simulink model "Full_Model_D_R2"  (R2013a)
settings: Solver=ode45  StartTime=0.0  StopTime=sim_length  MaxStep=1e-4  RelTol=1e-3
values from neighbouring files (symbols this model uses):
  B = 0    [Model_Parameters.mat]
  D = 4.45306861536e-07    [Model_Parameters.mat]
  F_yIntercept = -10.4432883127    [Model_Parameters.mat]
  Feed_Forward_Yaw_d = 0    [Yaw_Controller_SS_D_Data.mat]
  g = 9.81    [Model_Parameters.mat]
  I_Phi = I_Gamma    [Main_Controller_Test_C.m]
  I_Psi = 0.236966962973    [Model_Parameters.mat]
  I_Theta = 0.127422725814    [Model_Parameters.mat]
  J = 8e-08    [Model_Parameters.mat]
  Kf = 9.48907430341    [Model_Parameters.mat]
  Kw = 501.513336009    [Model_Parameters.mat]
  L = 0.338    [Model_Parameters.mat]
  Mass = 2.26    [Model_Parameters.mat]
  Motor_TimeConstant = 0.07    [Model_Parameters.mat]
  omega_0 = (5.6-F_yIntercept)/Kf    [Main_Controller_Test_C.m]
  omega_Lim = (0-F_yIntercept)/Kf    [Main_Controller_Test_C.m]
  Phi_IC = (2/180)*pi    (= 0.0349065850399)    [Main_Controller_Test_C.m]
  Pitch_Setpoint = 0    [Main_Controller_Test_C.m]
  Psi_IC = (10/180)*pi    (= 0.174532925199)    [Main_Controller_Test_C.m]
  PWM_IC = 1.4    [Main_Controller_Test_C.m]
  Speed_yIntercept = -347.939581678    [Model_Parameters.mat]
  Theta_IC = (2/180)*pi    (= 0.0349065850399)    [Main_Controller_Test_C.m]
  Yaw_Setpoint = 0    [Main_Controller_Test_C.m]
undefined symbols (not defined in the file or in its folder): DiscIntNeverNeededParam, Feed_Forward_Roll_d, Ts
libraries: simulink x6
settings Model: Creator=Ross  LastModifiedBy=Ross

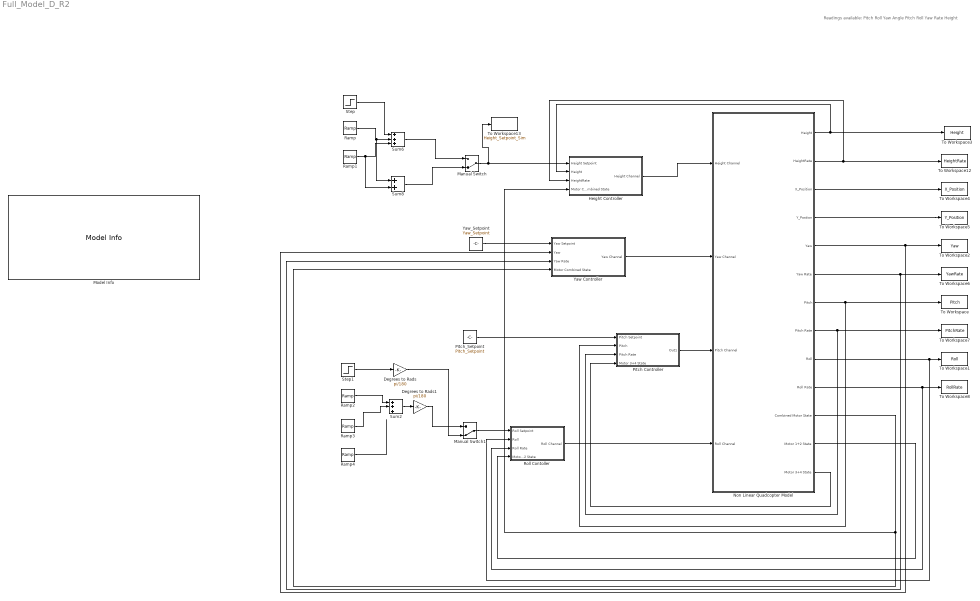
== system Full_Model_D_R2 ==
  note: Readings available:
      | Pitch Roll Yaw Angle
      | Pitch Roll Yaw Rate
      | Height
  Degrees to Rads : Gain  Gain=pi/180
  Degrees to Rads1 : Gain  Gain=pi/180
  Height Controller : Subsystem
  Manual Switch : ManualSwitch  CurrentSetting=0
  Manual Switch1 : ManualSwitch  CurrentSetting=0
  Model Info : simulink/Model-Wide Utilities/Model Info  InitialBlockCM=None  BlockCM=None  Frame=on  DisplayStringWithTags=|  HorizontalTextAlignment=Center  LeftAlignmentValue=0.5  SourceBlockDiagram=Full_Model_D_R2  TagMaxNumber=20
      | %<ModelName>
      | Simulink Diagram Used in Testing of Controllers designed for Quadcopters
      | Model version is %<ModelVersion>
      | 
      | %<Created>
      | %<ModifiedBy>
      | %<ModifiedDate>
      | %<ModifiedComment>
      | 
      | 
      | %<LastModifiedBy>
      | %<LastModificationDate>
      | %<Description>
  Non Linear Quadcopter Model : Subsystem
  Pitch Controller : Subsystem
  "Pitch_Setpoint " : Constant  Value=Pitch_Setpoint
  Ramp : simulink/Sources/Ramp  slope=1  start=2  X0=0
  Ramp1 : simulink/Sources/Ramp  slope=-1  start=5  X0=0
  Ramp2 : simulink/Sources/Ramp  slope=20  start=10  X0=0
  Ramp3 : simulink/Sources/Ramp  slope=-10  start=11  X0=0
  Ramp4 : simulink/Sources/Ramp  slope=2  start=22  X0=0
  Roll Contoller : Subsystem
  Step : Step  Time=10  SampleTime=0
  Step1 : Step  Time=12  After=40  SampleTime=0
  Sum2 : Sum  Inputs=+++
  Sum6 : Sum  Inputs=+++
  Sum8 : Sum
  To Workspace : ToWorkspace  VariableName=Pitch  SampleTime=-1  SaveFormat=Timeseries
  To Workspace1 : ToWorkspace  VariableName=Roll  SampleTime=-1  SaveFormat=Timeseries
  To Workspace12 : ToWorkspace  VariableName=HeightRate  SampleTime=-1  SaveFormat=Timeseries
  To Workspace13 : ToWorkspace  VariableName=Height_Setpoint_Sim  SampleTime=-1  SaveFormat=Timeseries
  To Workspace2 : ToWorkspace  VariableName=Yaw  SampleTime=-1  SaveFormat=Timeseries
  To Workspace3 : ToWorkspace  VariableName=Height  SampleTime=-1  SaveFormat=Timeseries
  To Workspace4 : ToWorkspace  VariableName=X_Position  SampleTime=-1  SaveFormat=Timeseries
  To Workspace5 : ToWorkspace  VariableName=Y_Position  SampleTime=-1  SaveFormat=Timeseries
  To Workspace6 : ToWorkspace  VariableName=YawRate  SampleTime=-1  SaveFormat=Timeseries
  To Workspace7 : ToWorkspace  VariableName=PitchRate  SampleTime=-1  SaveFormat=Timeseries
  To Workspace8 : ToWorkspace  VariableName=RollRate  SampleTime=-1  SaveFormat=Timeseries
  Yaw Controller : Subsystem
  Yaw_Setpoint : Constant  Value=Yaw_Setpoint
  wires:
  Non Linear Quadcopter Model/5(Yaw) -> Yaw Controller/2(Yaw), To Workspace2/1
  Non Linear Quadcopter Model/1(Height) -> To Workspace3/1, Height Controller/2(Height)
  Non Linear Quadcopter Model/3(X_Position) -> To Workspace4/1
  Non Linear Quadcopter Model/4(Y_Postion) -> To Workspace5/1
  Non Linear Quadcopter Model/6(Yaw Rate) -> Yaw Controller/3(Yaw Rate), To Workspace6/1
  Non Linear Quadcopter Model/8(Pitch Rate) -> Pitch Controller/3(Pitch Rate), To Workspace7/1
  Non Linear Quadcopter Model/10(Roll Rate) -> To Workspace8/1, Roll Contoller/3(Roll Rate)
  Ramp/1 -> Sum8/1, Sum6/2
  Ramp1/1 -> Sum8/2, Sum6/3
  Step/1 -> Sum6/1
  Manual Switch/1 -> Height Controller/1(Height Setpoint), To Workspace13/1
  Sum8/1 -> Manual Switch/2
  Sum6/1 -> Manual Switch/1
  Non Linear Quadcopter Model/9(Roll) -> To Workspace1/1, Roll Contoller/2(Roll)
  Non Linear Quadcopter Model/7(Pitch) -> Pitch Controller/2(Pitch), To Workspace/1
  Ramp2/1 -> Sum2/1
  Ramp3/1 -> Sum2/2
  Step1/1 -> Degrees to Rads/1
  Sum2/1 -> Degrees to Rads1/1
  Degrees to Rads/1 -> Manual Switch1/2
  "Pitch_Setpoint "/1 -> Pitch Controller/1(Pitch Setpoint)
  Non Linear Quadcopter Model/13(Motor 3+4 State) -> Pitch Controller/4(Motor 3+4 State)
  Pitch Controller/1(Out1) -> Non Linear Quadcopter Model/3(Pitch Channel)
  Manual Switch1/1 -> Roll Contoller/1("Roll Setpoint ")
  Non Linear Quadcopter Model/12(Motor 1+2 State) -> Roll Contoller/4(Motor 1+2 State)
  Roll Contoller/1(Roll Channel) -> Non Linear Quadcopter Model/4(Roll Channel)
  Yaw_Setpoint/1 -> Yaw Controller/1(Yaw Setpoint)
  Yaw Controller/1(Yaw Channel) -> Non Linear Quadcopter Model/2(Yaw Channel)
  Height Controller/1(Height Channel) -> Non Linear Quadcopter Model/1(Height Channel)
  Non Linear Quadcopter Model/2(HeightRate) -> Height Controller/3(HeightRate), To Workspace12/1
  Non Linear Quadcopter Model/11(Combined Motor State) -> Height Controller/4(Motor Combined State), Yaw Controller/4(Motor Combined State)
  Degrees to Rads1/1 -> Manual Switch1/1
  Ramp4/1 -> ?

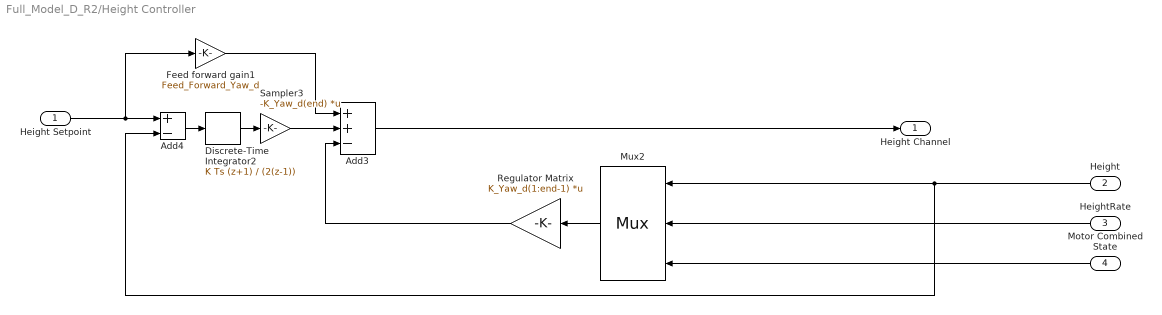
== system Full_Model_D_R2/Height Controller ==
  Height Setpoint : Inport
  Height : Inport  Port=2
  HeightRate : Inport  Port=3
  Motor Combined State : Inport  Port=4
  Add3 : Sum  Inputs=++-
  Add4 : Sum  Inputs=+-  SampleTime=Ts
  Discrete-Time Integrator2 : DiscreteIntegrator  IntegratorMethod=Integration: Trapezoidal  gainval=1  InitialCondition=PWM_IC  SampleTime=Ts  ICPrevOutput=DiscIntNeverNeededParam  ICPrevScaledInput=DiscIntNeverNeededParam
  Feed forward gain1 : Gain  Gain=Feed_Forward_Yaw_d  SampleTime=Ts
  Mux2 : Mux  Inputs=3
      settings: DisplayOption=signals
  Regulator Matrix : Gain  Gain=K_Yaw_d(1:end-1)  Multiplication=Matrix(K*u)  SampleTime=Ts
  Sampler3 : Gain  Gain=-K_Yaw_d(end)  Multiplication=Matrix(K*u)  SampleTime=Ts
  Height Channel : Outport
  wires:
  Height/1 -> Add4/2, Mux2/1
  Feed forward gain1/1 -> Add3/1
  Add3/1 -> Height Channel/1
  Motor Combined State/1 -> Mux2/3
  Mux2/1 -> Regulator Matrix/1
  Regulator Matrix/1 -> Add3/3
  Add4/1 -> Discrete-Time Integrator2/1
  Discrete-Time Integrator2/1 -> Sampler3/1
  Sampler3/1 -> Add3/2
  Height Setpoint/1 -> Feed forward gain1/1, Add4/1
  HeightRate/1 -> Mux2/2

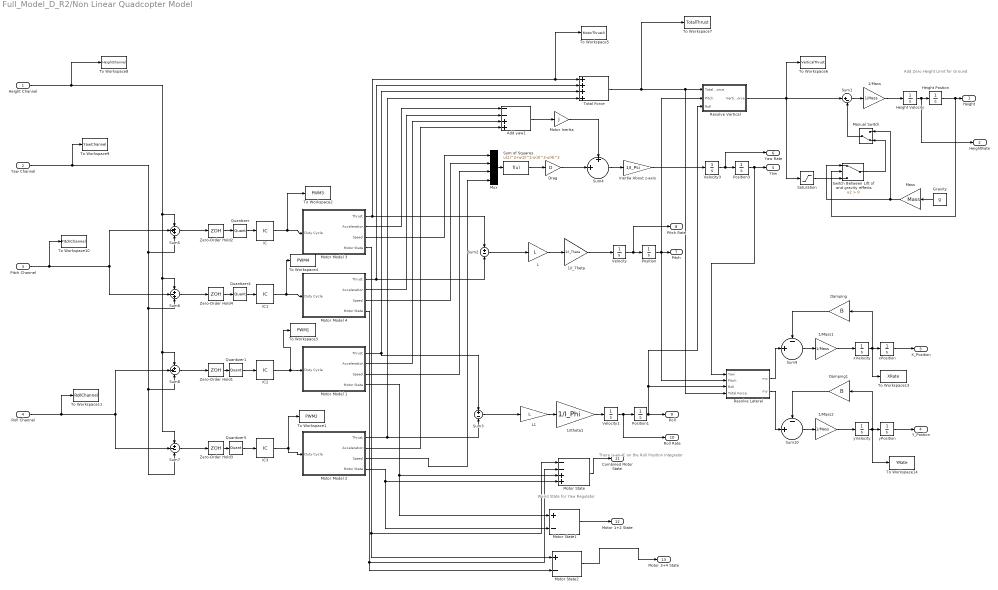
== system Full_Model_D_R2/Non Linear Quadcopter Model ==
  note: Weird State for Yaw
      | Regulator
  note: There is an IC on the Roll
      | Position Integrator
  note: Add Zero Height Limit
      | for Ground
  Height Channel : Inport
  Yaw Channel : Inport  Port=2
  Pitch Channel : Inport  Port=3
  Roll Channel : Inport  Port=4
  1/I_Theta : Gain  Gain=1/I_Theta
  1/Itheta1 : Gain  Gain=1/I_Phi
  1/Mass : Gain  Gain=1/Mass
  1/Mass1 : Gain  Gain=1/Mass
  1/Mass2 : Gain  Gain=1/Mass
  Add yaw1 : Sum  Inputs=--++
  Damping : Gain  Gain=B
  Damping1 : Gain  Gain=B
  Drag : Gain  Gain=D
  Gravity : Constant  Value=g
  Height Postion : Integrator  LowerSaturationLimit=0
  Height Velocity : Integrator
  IC{,1..3} (4 alike) : InitialCondition
  Inertia About z-axis : Gain  Gain=1/I_Psi
  L : Gain  Gain=L
  L1 : Gain  Gain=L
  Manual Switch : ManualSwitch  CurrentSetting=0
  Mass : Gain  Gain=Mass
  Motor Inertia : Gain  Gain=J
  Motor Model 1 : Subsystem
  Motor Model 2 : Subsystem
  Motor Model 3 : Subsystem
  Motor Model 4 : Subsystem
  Motor State : Sum  Inputs=--++
  Motor State1 : Sum  Inputs=+-
  Motor State2 : Sum  Inputs=+-
  Mux : Mux
  Position : Integrator  InitialCondition=Theta_IC
  Position1 : Integrator  InitialCondition=Phi_IC
  Position3 : Integrator  InitialCondition=Psi_IC
  Quantizer{,1,4..5} (4 alike) : Quantizer  QuantizationInterval=8.2e-3
  Resolve Lateral : Subsystem
  Resolve Vertical : Subsystem
  Saturation : Saturate  UpperLimit=Mass*g  LowerLimit=-inf
  Sum of Squares : Fcn  Expr=u(1)^2+u(2)^2-u(3)^2-u(4)^2
  Sum1 : Sum  Inputs=|+-
  Sum10 : Sum  Inputs=-|||+||||
  Sum2 : Sum  Inputs=+|-
  Sum3 : Sum  Inputs=+|-
  Sum4 : Sum  Inputs=+|||+||||
  Sum5 : Sum  Inputs=+++
  Sum6 : Sum  Inputs=+-+
  Sum7 : Sum  Inputs=+--
  Sum8 : Sum  Inputs=++-
  Sum9 : Sum  Inputs=-|||+||||
  Switch Between Lift of and gravity effects : Switch  Criteria=u2 > Threshold
  To Workspace1 : ToWorkspace  VariableName=PWM2  SampleTime=-1  SaveFormat=Timeseries
  To Workspace10 : ToWorkspace  VariableName=PitchChannel  SampleTime=-1  SaveFormat=Timeseries
  To Workspace11 : ToWorkspace  VariableName=RollChannel  SampleTime=-1  SaveFormat=Timeseries
  To Workspace13 : ToWorkspace  VariableName=XRate  SampleTime=-1  SaveFormat=Timeseries
  To Workspace14 : ToWorkspace  VariableName=YRate  SampleTime=-1  SaveFormat=Timeseries
  To Workspace2 : ToWorkspace  VariableName=PWM3  SampleTime=-1  SaveFormat=Timeseries
  To Workspace3 : ToWorkspace  VariableName=PWM1  SampleTime=-1  SaveFormat=Timeseries
  To Workspace4 : ToWorkspace  VariableName=PWM4  SampleTime=-1  SaveFormat=Timeseries
  To Workspace5 : ToWorkspace  VariableName=MotorThrust3  SampleTime=-1  SaveFormat=Timeseries
  To Workspace6 : ToWorkspace  VariableName=VerticalThrust  SampleTime=-1  SaveFormat=Timeseries
  To Workspace7 : ToWorkspace  VariableName=TotalThrust  SampleTime=-1  SaveFormat=Timeseries
  To Workspace8 : ToWorkspace  VariableName=HeightChannel  SampleTime=-1  SaveFormat=Timeseries
  To Workspace9 : ToWorkspace  VariableName=YawChannel  SampleTime=-1  SaveFormat=Timeseries
  Total Force : Sum  Inputs=++++
  Velocity : Integrator
  Velocity1 : Integrator
  Velocity3 : Integrator
  Zero-Order Hold{1..4} (4 alike) : ZeroOrderHold  SampleTime=Ts
  xPosition : Integrator
  xVelocity : Integrator
  yPosition : Integrator
  yVelocity : Integrator
  Height : Outport
  HeightRate : Outport  Port=2
  X_Position : Outport  Port=3
  Y_Postion : Outport  Port=4
  Yaw : Outport  Port=5
  Yaw Rate : Outport  Port=6
  Pitch : Outport  Port=7
  Pitch Rate : Outport  Port=8
  Roll : Outport  Port=9
  Roll Rate : Outport  Port=10
  Combined Motor State : Outport  Port=11
  Motor 1+2 State : Outport  Port=12
  Motor 3+4 State : Outport  Port=13
  wires:
  Sum1/1 -> 1/Mass/1
  Pitch Channel/1 -> Sum6/2, Sum5/2, To Workspace10/1
  Add yaw1/1 -> Motor Inertia/1
  1/Mass/1 -> Height Velocity/1
  Motor Inertia/1 -> Sum4/1
  1/Mass1/1 -> xVelocity/1
  Sum9/1 -> 1/Mass1/1
  xPosition/1 -> X_Position/1
  Damping/1 -> Sum9/1
  xVelocity/1 -> To Workspace13/1, Damping/1, xPosition/1
  Motor Model 3/2(Acceleration) -> Add yaw1/1
  Height Velocity/1 -> HeightRate/1, Height Postion/1
  Sum2/1 -> L/1
  1/I_Theta/1 -> Velocity/1
  Velocity/1 -> Pitch Rate/1, Position/1
  Position/1 -> Resolve Vertical/2(Pitch), Pitch/1, Resolve Lateral/2(Pitch)
  Total Force/1 -> To Workspace7/1, Resolve Lateral/4(Total Force), Resolve Vertical/1(Total Force)
  Sum of Squares/1 -> Drag/1
  Drag/1 -> Sum4/2
  Position3/1 -> Yaw/1, Resolve Lateral/1(Yaw)
  Velocity3/1 -> Yaw Rate/1, Position3/1
  Inertia About z-axis/1 -> Velocity3/1
  Motor Model 2/1(Thrust) -> Total Force/4, Sum3/2
  L1/1 -> 1/Itheta1/1
  Velocity1/1 -> Roll Rate/1, Position1/1
  Sum3/1 -> L1/1
  Position1/1 -> Roll/1, Resolve Lateral/3(Roll), Resolve Vertical/3(Roll)
  1/Itheta1/1 -> Velocity1/1
  Motor Model 3/1(Thrust) -> Sum2/1, To Workspace5/1, Total Force/1
  Sum10/1 -> 1/Mass2/1
  1/Mass2/1 -> yVelocity/1
  yPosition/1 -> Y_Postion/1
  Damping1/1 -> Sum10/1
  yVelocity/1 -> Damping1/1, To Workspace14/1, yPosition/1
  Height Postion/1 -> Switch Between Lift of and gravity effects/2, Height/1
  Motor Model 1/2(Acceleration) -> Add yaw1/3
  Motor Model 4/1(Thrust) -> Sum2/2, Total Force/2
  Sum4/1 -> Inertia About z-axis/1
  Motor Model 1/1(Thrust) -> Sum3/1, Total Force/3
  Height Channel/1 -> To Workspace8/1, Sum6/1, Sum7/1, Sum8/1, Sum5/1
  Yaw Channel/1 -> To Workspace9/1, Sum7/3, Sum8/3, Sum6/3, Sum5/3
  Motor Model 4/2(Acceleration) -> Add yaw1/2
  Motor Model 2/2(Acceleration) -> Add yaw1/4
  Roll Channel/1 -> To Workspace11/1, Sum8/2, Sum7/2
  Gravity/1 -> Mass/1
  Resolve Lateral/1(mx) -> Sum9/2
  Resolve Lateral/2(my) -> Sum10/2
  Motor Model 3/3(Speed) -> Mux/1
  Motor Model 4/3(Speed) -> Mux/2
  Motor Model 1/3(Speed) -> Mux/3
  Motor Model 2/3(Speed) -> Mux/4
  Mux/1 -> Sum of Squares/1
  L/1 -> 1/I_Theta/1
  Switch Between Lift of and gravity effects/1 -> Manual Switch/2
  Saturation/1 -> Switch Between Lift of and gravity effects/3
  Mass/1 -> Manual Switch/1, Switch Between Lift of and gravity effects/1
  Manual Switch/1 -> Sum1/2
  Motor Model 3/4(Motor State) -> Motor State2/1, Motor State/1
  Motor Model 4/4(Motor State) -> Motor State2/2, Motor State/2
  Motor Model 1/4(Motor State) -> Motor State1/1, Motor State/3
  Motor Model 2/4(Motor State) -> Motor State1/2, Motor State/4
  Motor State/1 -> Combined Motor State/1
  Motor State1/1 -> Motor 1+2 State/1
  Motor State2/1 -> Motor 3+4 State/1
  Resolve Vertical/1(Vertical Force) -> Sum1/1, Saturation/1, To Workspace6/1
  Zero-Order Hold2/1 -> Quantizer/1
  Zero-Order Hold1/1 -> Quantizer1/1
  Zero-Order Hold3/1 -> Quantizer5/1
  Zero-Order Hold4/1 -> Quantizer4/1
  IC1/1 -> To Workspace4/1, Motor Model 4/1(Duty Cycle)
  IC2/1 -> To Workspace3/1, Motor Model 1/1(Duty Cycle)
  IC3/1 -> Motor Model 2/1(Duty Cycle), To Workspace1/1
  IC/1 -> To Workspace2/1, Motor Model 3/1(Duty Cycle)
  Sum5/1 -> Zero-Order Hold2/1
  Sum6/1 -> Zero-Order Hold4/1
  Sum8/1 -> Zero-Order Hold1/1
  Sum7/1 -> Zero-Order Hold3/1
  Quantizer/1 -> IC/1
  Quantizer4/1 -> IC1/1
  Quantizer1/1 -> IC2/1
  Quantizer5/1 -> IC3/1

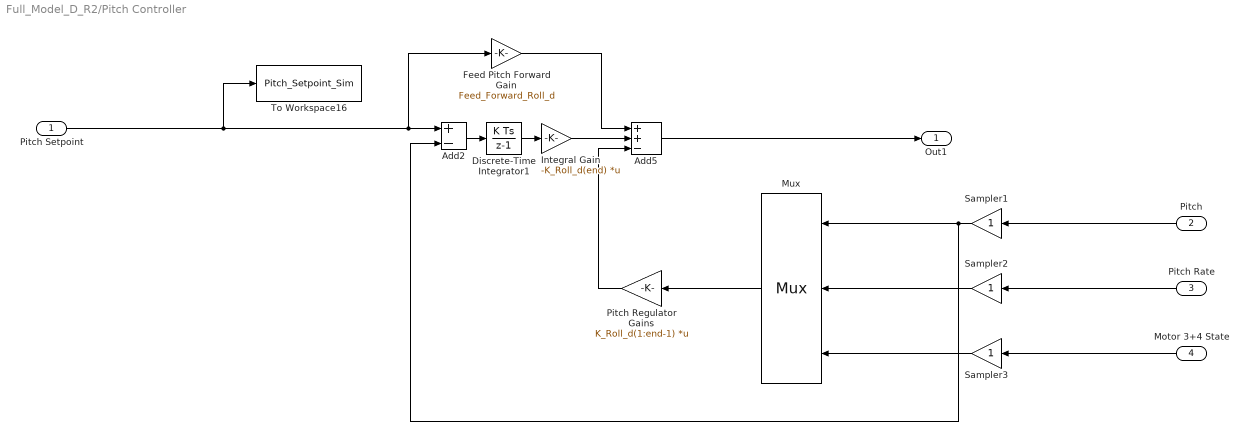
== system Full_Model_D_R2/Pitch Controller ==
  Pitch Setpoint : Inport
  Pitch : Inport  Port=2
  Pitch Rate : Inport  Port=3
  Motor 3+4 State : Inport  Port=4
  Add2 : Sum  Inputs=+-
  Add5 : Sum  Inputs=++-
  Discrete-Time Integrator1 : DiscreteIntegrator  gainval=1  InitialCondition=PWM_IC  SampleTime=Ts  ICPrevOutput=DiscIntNeverNeededParam  ICPrevScaledInput=DiscIntNeverNeededParam
  Feed Pitch Forward Gain : Gain  Gain=Feed_Forward_Roll_d  SampleTime=Ts
  Integral Gain : Gain  Gain=-K_Roll_d(end)  Multiplication=Matrix(K*u)  SampleTime=Ts
  Mux : Mux  Inputs=3
      settings: DisplayOption=signals
  Pitch Regulator Gains : Gain  Gain=K_Roll_d(1:end-1)  Multiplication=Matrix(K*u)
  Sampler1 : Gain  SampleTime=Ts
  Sampler2 : Gain  SampleTime=Ts
  Sampler3 : Gain  SampleTime=Ts
  To Workspace16 : ToWorkspace  VariableName=Pitch_Setpoint_Sim  SampleTime=-1  SaveFormat=Timeseries
  Out1 : Outport
  wires:
  Integral Gain/1 -> Add5/2
  Sampler1/1 -> Add2/2, Mux/1
  Pitch Setpoint/1 -> To Workspace16/1, Feed Pitch Forward Gain/1, Add2/1
  Sampler2/1 -> Mux/2
  Discrete-Time Integrator1/1 -> Integral Gain/1
  Add2/1 -> Discrete-Time Integrator1/1
  Sampler3/1 -> Mux/3
  Add5/1 -> Out1/1
  Mux/1 -> Pitch Regulator Gains/1
  Pitch Regulator Gains/1 -> Add5/3
  Motor 3+4 State/1 -> Sampler3/1
  Feed Pitch Forward Gain/1 -> Add5/1
  Pitch Rate/1 -> Sampler2/1
  Pitch/1 -> Sampler1/1

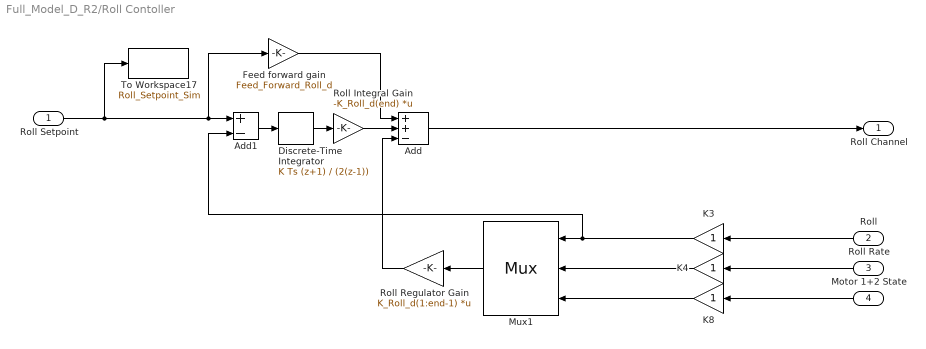
== system Full_Model_D_R2/Roll Contoller ==
  "Roll Setpoint " : Inport
  Roll : Inport  Port=2
  Roll Rate : Inport  Port=3
  Motor 1+2 State : Inport  Port=4
  Add : Sum  Inputs=++-
  Add1 : Sum  Inputs=+-
  Discrete-Time Integrator : DiscreteIntegrator  IntegratorMethod=Integration: Trapezoidal  gainval=1  InitialCondition=PWM_IC  SampleTime=Ts  ICPrevOutput=DiscIntNeverNeededParam  ICPrevScaledInput=DiscIntNeverNeededParam
  Feed forward gain : Gain  Gain=Feed_Forward_Roll_d  SampleTime=Ts
  K3 : Gain  SampleTime=Ts
  K4 : Gain  SampleTime=Ts
  K8 : Gain  SampleTime=Ts
  Mux1 : Mux  Inputs=3
      settings: DisplayOption=signals
  Roll Integral Gain : Gain  Gain=-K_Roll_d(end)  Multiplication=Matrix(K*u)  SampleTime=Ts
  Roll Regulator Gain : Gain  Gain=K_Roll_d(1:end-1)  Multiplication=Matrix(K*u)
  To Workspace17 : ToWorkspace  VariableName=Roll_Setpoint_Sim  SampleTime=-1  SaveFormat=Timeseries
  Roll Channel : Outport
  wires:
  Roll/1 -> K3/1
  K4/1 -> Mux1/2
  K8/1 -> Mux1/3
  Add1/1 -> Discrete-Time Integrator/1
  Discrete-Time Integrator/1 -> Roll Integral Gain/1
  Roll Integral Gain/1 -> Add/2
  K3/1 -> Add1/2, Mux1/1
  "Roll Setpoint "/1 -> Feed forward gain/1, Add1/1, To Workspace17/1
  Feed forward gain/1 -> Add/1
  Roll Regulator Gain/1 -> Add/3
  Mux1/1 -> Roll Regulator Gain/1
  Motor 1+2 State/1 -> K8/1
  Add/1 -> Roll Channel/1
  Roll Rate/1 -> K4/1

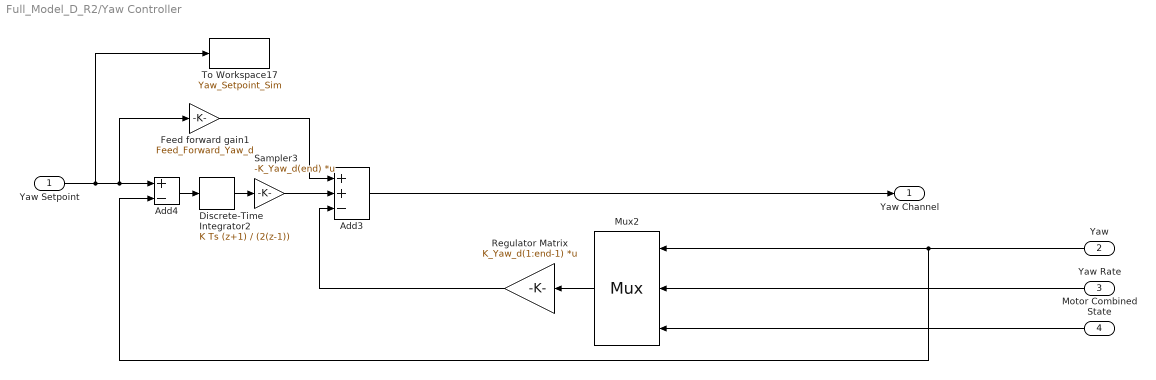
== system Full_Model_D_R2/Yaw Controller ==
  Yaw Setpoint : Inport
  Yaw : Inport  Port=2
  Yaw Rate : Inport  Port=3
  Motor Combined State : Inport  Port=4
  Add3 : Sum  Inputs=++-
  Add4 : Sum  Inputs=+-  SampleTime=Ts
  Discrete-Time Integrator2 : DiscreteIntegrator  IntegratorMethod=Integration: Trapezoidal  gainval=1  InitialCondition=PWM_IC  SampleTime=Ts  ICPrevOutput=DiscIntNeverNeededParam  ICPrevScaledInput=DiscIntNeverNeededParam
  Feed forward gain1 : Gain  Gain=Feed_Forward_Yaw_d  SampleTime=Ts
  Mux2 : Mux  Inputs=3
      settings: DisplayOption=signals
  Regulator Matrix : Gain  Gain=K_Yaw_d(1:end-1)  Multiplication=Matrix(K*u)  SampleTime=Ts
  Sampler3 : Gain  Gain=-K_Yaw_d(end)  Multiplication=Matrix(K*u)  SampleTime=Ts
  To Workspace17 : ToWorkspace  VariableName=Yaw_Setpoint_Sim  SampleTime=-1  SaveFormat=Timeseries
  Yaw Channel : Outport
  wires:
  Yaw/1 -> Add4/2, Mux2/1
  Feed forward gain1/1 -> Add3/1
  Add3/1 -> Yaw Channel/1
  Motor Combined State/1 -> Mux2/3
  Mux2/1 -> Regulator Matrix/1
  Regulator Matrix/1 -> Add3/3
  Add4/1 -> Discrete-Time Integrator2/1
  Discrete-Time Integrator2/1 -> Sampler3/1
  Sampler3/1 -> Add3/2
  Yaw Setpoint/1 -> To Workspace17/1, Feed forward gain1/1, Add4/1
  Yaw Rate/1 -> Mux2/2

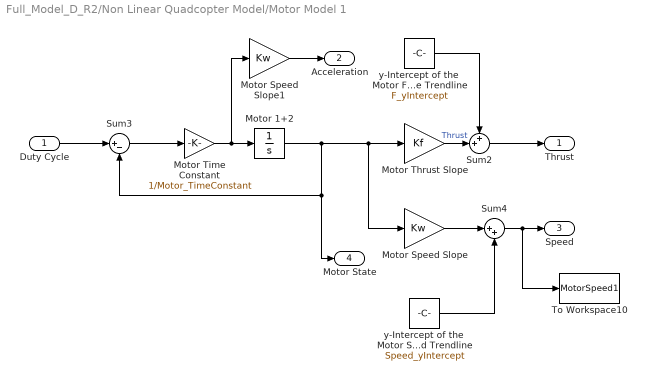
== system Full_Model_D_R2/Non Linear Quadcopter Model/Motor Model 1 ==
  Duty Cycle : Inport
  Motor 1+2 : Integrator  InitialCondition=omega_0  LimitOutput=on  LowerSaturationLimit=omega_Lim
  Motor Speed Slope : Gain  Gain=Kw
  Motor Speed Slope1 : Gain  Gain=Kw
  Motor Thrust Slope : Gain  Gain=Kf
  Motor Time Constant : Gain  Gain=1/Motor_TimeConstant
  Sum2 : Sum  Inputs=++|
  Sum3 : Sum  Inputs=|+-
  Sum4 : Sum  Inputs=|++
  To Workspace10 : ToWorkspace  VariableName=MotorSpeed1  SampleTime=-1  SaveFormat=Timeseries
  y-Intercept of the  Motor Force Trendline : Constant  Value=F_yIntercept
  y-Intercept of the  Motor Speed Trendline : Constant  Value=Speed_yIntercept
  Thrust : Outport
  Acceleration : Outport  Port=2
  Speed : Outport  Port=3
  Motor State : Outport  Port=4
  wires:
  Motor Thrust Slope/1 -> Sum2/2  "Thrust"
  Motor 1+2/1 -> Motor State/1, Sum3/2, Motor Speed Slope/1, Motor Thrust Slope/1
  Duty Cycle/1 -> Sum3/1
  Sum3/1 -> Motor Time Constant/1
  Motor Time Constant/1 -> Motor 1+2/1, Motor Speed Slope1/1
  Motor Speed Slope/1 -> Sum4/1
  Motor Speed Slope1/1 -> Acceleration/1
  Sum2/1 -> Thrust/1
  y-Intercept of the  Motor Force Trendline/1 -> Sum2/1
  Sum4/1 -> To Workspace10/1, Speed/1
  y-Intercept of the  Motor Speed Trendline/1 -> Sum4/2

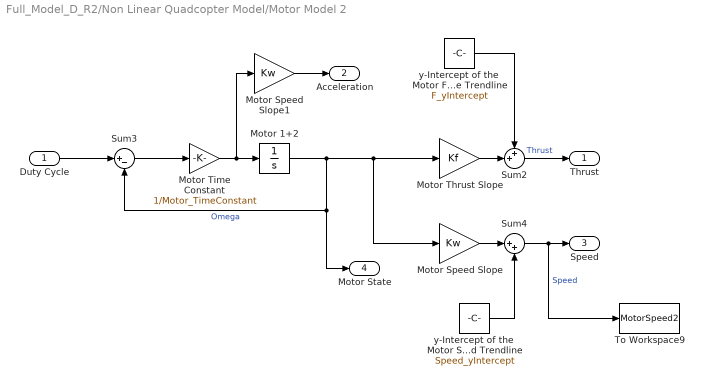
== system Full_Model_D_R2/Non Linear Quadcopter Model/Motor Model 2 ==
  Duty Cycle : Inport
  Motor 1+2 : Integrator  InitialCondition=omega_0  LimitOutput=on  LowerSaturationLimit=omega_Lim
  Motor Speed Slope : Gain  Gain=Kw
  Motor Speed Slope1 : Gain  Gain=Kw
  Motor Thrust Slope : Gain  Gain=Kf
  Motor Time Constant : Gain  Gain=1/Motor_TimeConstant
  Sum2 : Sum  Inputs=++|
  Sum3 : Sum  Inputs=|+-
  Sum4 : Sum  Inputs=|++
  To Workspace9 : ToWorkspace  VariableName=MotorSpeed2  SampleTime=-1  SaveFormat=Timeseries
  y-Intercept of the  Motor Force Trendline : Constant  Value=F_yIntercept
  y-Intercept of the  Motor Speed Trendline : Constant  Value=Speed_yIntercept
  Thrust : Outport
  Acceleration : Outport  Port=2
  Speed : Outport  Port=3
  Motor State : Outport  Port=4
  wires:
  Motor Thrust Slope/1 -> Sum2/2
  Motor 1+2/1 -> Sum3/2, Motor State/1, Motor Speed Slope/1, Motor Thrust Slope/1  "Omega"
  Duty Cycle/1 -> Sum3/1
  Sum3/1 -> Motor Time Constant/1
  Motor Time Constant/1 -> Motor 1+2/1, Motor Speed Slope1/1
  Motor Speed Slope/1 -> Sum4/1
  Motor Speed Slope1/1 -> Acceleration/1
  Sum2/1 -> Thrust/1  "Thrust"
  y-Intercept of the  Motor Force Trendline/1 -> Sum2/1
  Sum4/1 -> To Workspace9/1, Speed/1  "Speed"
  y-Intercept of the  Motor Speed Trendline/1 -> Sum4/2

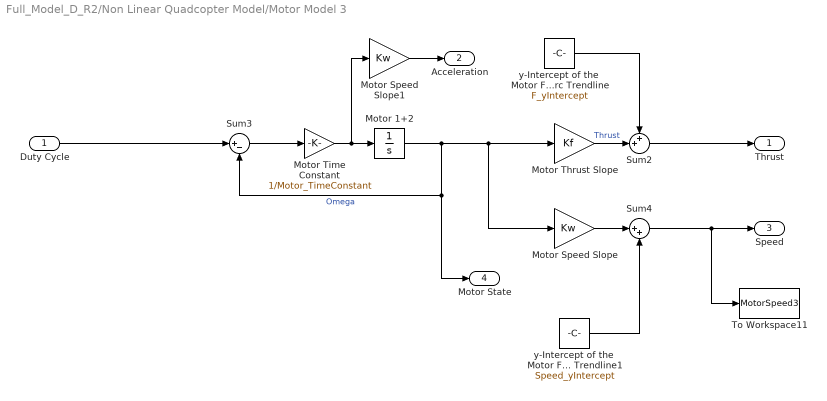
== system Full_Model_D_R2/Non Linear Quadcopter Model/Motor Model 3 ==
  Duty Cycle : Inport
  Motor 1+2 : Integrator  InitialCondition=omega_0  LimitOutput=on  LowerSaturationLimit=omega_Lim
  Motor Speed Slope : Gain  Gain=Kw
  Motor Speed Slope1 : Gain  Gain=Kw
  Motor Thrust Slope : Gain  Gain=Kf
  Motor Time Constant : Gain  Gain=1/Motor_TimeConstant
  Sum2 : Sum  Inputs=++|
  Sum3 : Sum  Inputs=|+-
  Sum4 : Sum  Inputs=|++
  To Workspace11 : ToWorkspace  VariableName=MotorSpeed3  SampleTime=-1  SaveFormat=Timeseries
  y-Intercept of the  Motor Forc Trendline : Constant  Value=F_yIntercept
  y-Intercept of the  Motor Forc Trendline1 : Constant  Value=Speed_yIntercept
  Thrust : Outport
  Acceleration : Outport  Port=2
  Speed : Outport  Port=3
  Motor State : Outport  Port=4
  wires:
  Motor Thrust Slope/1 -> Sum2/2  "Thrust"
  Motor 1+2/1 -> Motor State/1, Sum3/2, Motor Speed Slope/1, Motor Thrust Slope/1  "Omega"
  Duty Cycle/1 -> Sum3/1
  Sum3/1 -> Motor Time Constant/1
  Motor Time Constant/1 -> Motor 1+2/1, Motor Speed Slope1/1
  Motor Speed Slope/1 -> Sum4/1
  Motor Speed Slope1/1 -> Acceleration/1
  y-Intercept of the  Motor Forc Trendline/1 -> Sum2/1
  y-Intercept of the  Motor Forc Trendline1/1 -> Sum4/2
  Sum2/1 -> Thrust/1
  Sum4/1 -> To Workspace11/1, Speed/1

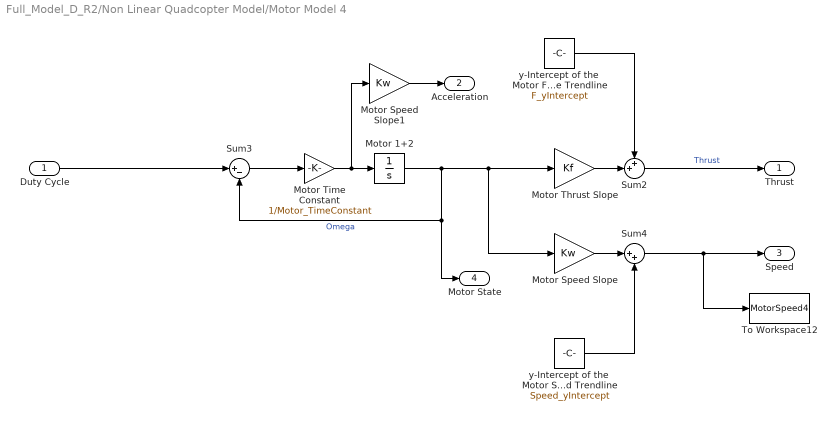
== system Full_Model_D_R2/Non Linear Quadcopter Model/Motor Model 4 ==
  Duty Cycle : Inport
  Motor 1+2 : Integrator  InitialCondition=omega_0  LimitOutput=on  LowerSaturationLimit=omega_Lim
  Motor Speed Slope : Gain  Gain=Kw
  Motor Speed Slope1 : Gain  Gain=Kw
  Motor Thrust Slope : Gain  Gain=Kf
  Motor Time Constant : Gain  Gain=1/Motor_TimeConstant
  Sum2 : Sum  Inputs=++|
  Sum3 : Sum  Inputs=|+-
  Sum4 : Sum  Inputs=|++
  To Workspace12 : ToWorkspace  VariableName=MotorSpeed4  SampleTime=-1  SaveFormat=Timeseries
  y-Intercept of the  Motor Force Trendline : Constant  Value=F_yIntercept
  y-Intercept of the  Motor Speed Trendline : Constant  Value=Speed_yIntercept
  Thrust : Outport
  Acceleration : Outport  Port=2
  Speed : Outport  Port=3
  Motor State : Outport  Port=4
  wires:
  Motor Thrust Slope/1 -> Sum2/2
  Motor 1+2/1 -> Motor State/1, Sum3/2, Motor Speed Slope/1, Motor Thrust Slope/1  "Omega"
  Duty Cycle/1 -> Sum3/1
  Sum3/1 -> Motor Time Constant/1
  Motor Time Constant/1 -> Motor 1+2/1, Motor Speed Slope1/1
  Motor Speed Slope/1 -> Sum4/1
  Motor Speed Slope1/1 -> Acceleration/1
  Sum2/1 -> Thrust/1  "Thrust"
  y-Intercept of the  Motor Force Trendline/1 -> Sum2/1
  y-Intercept of the  Motor Speed Trendline/1 -> Sum4/2
  Sum4/1 -> To Workspace12/1, Speed/1

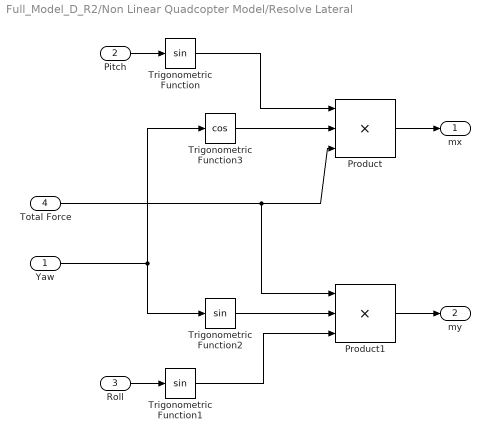
== system Full_Model_D_R2/Non Linear Quadcopter Model/Resolve Lateral ==
  Yaw : Inport
  Pitch : Inport  Port=2
  Roll : Inport  Port=3
  Total Force : Inport  Port=4
  Product : Product  Inputs=3
  Product1 : Product  Inputs=3
  Trigonometric Function : Trigonometry
  Trigonometric Function1 : Trigonometry
  Trigonometric Function2 : Trigonometry
  Trigonometric Function3 : Trigonometry  Operator=cos
  mx : Outport
  my : Outport  Port=2
  wires:
  Trigonometric Function/1 -> Product/1
  Total Force/1 -> Product1/1, Product/3
  Product/1 -> mx/1
  Roll/1 -> Trigonometric Function1/1
  Trigonometric Function1/1 -> Product1/3
  Product1/1 -> my/1
  Trigonometric Function3/1 -> Product/2
  Trigonometric Function2/1 -> Product1/2
  Yaw/1 -> Trigonometric Function2/1, Trigonometric Function3/1
  Pitch/1 -> Trigonometric Function/1

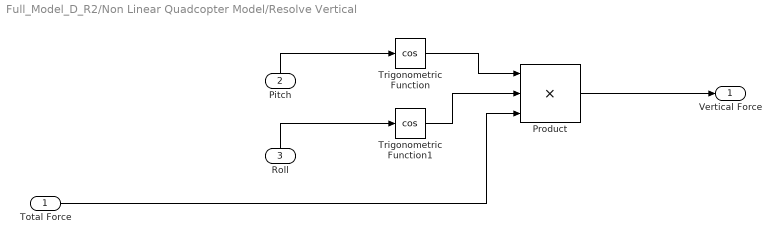
== system Full_Model_D_R2/Non Linear Quadcopter Model/Resolve Vertical ==
  Total Force : Inport
  Pitch : Inport  Port=2
  Roll : Inport  Port=3
  Product : Product  Inputs=3
  Trigonometric Function : Trigonometry  Operator=cos
  Trigonometric Function1 : Trigonometry  Operator=cos
  Vertical Force : Outport
  wires:
  Trigonometric Function/1 -> Product/1
  Total Force/1 -> Product/3
  Roll/1 -> Trigonometric Function1/1
  Pitch/1 -> Trigonometric Function/1
  Product/1 -> Vertical Force/1
  Trigonometric Function1/1 -> Product/2
